simulink model "Code_Gen_Model"  (R2023b)
settings: Solver=FixedStepDiscrete  StartTime=0.0  StopTime=inf  FixedStep=t_sample  RelTol=1e-3
settings Model: Creator=FIRSTMentor  LastModifiedBy=USER
settings OptimizationCC: DefaultParameterBehavior=Inlined  StrengthReduction=on  PassReuseOutputArgsAs=Individual arguments  ZeroExternalMemoryAtStartup=off  ZeroInternalMemoryAtStartup=off  OptimizeBlockOrder=speed  OptimizationPriority=Speed  OptimizationCustomize=off  MultiThreadedLoops=on  EfficientTunableParamExpr=on
settings DebuggingCC: MergeDetectMultiDrivingBlocksExec=none  ParameterTunabilityLossMsg=error
settings HardwareCC: ProdBitPerPointer=32  ProdBitPerSizeT=32  ProdBitPerPtrDiffT=32  ProdLargestAtomicInteger=Long  ProdWordSize=32  ProdHWDeviceType=ARM Compatible->ARM 7
settings ModelReferenceCC: PropagateSignalLabelsOutOfModel=off
settings SFSimCC: MATLABDynamicMemAlloc=off
settings RTWCC: Description=Embedded Coder  SystemTargetFile=ert.tlc  GenCodeOnly=on  TemplateMakefile=ert_default_tmf  Toolchain=MinGW64 | gmake (64-bit Windows)
settings CodeAppCC: ForceParamTrailComments=on  IgnoreCustomStorageClasses=off  OperatorAnnotations=on  SimulinkDataObjDesc=on  SFDataObjDesc=on  InsertBlockDesc=on
settings ERTTargetCC: TargetLangStandard=C99 (ISO)  SupportVariableSizeSignals=on  ParenthesesLevel=Maximum  InlinedParameterPlacement=NonHierarchical  ERTCustomFileTemplate=example_file_process.tlc

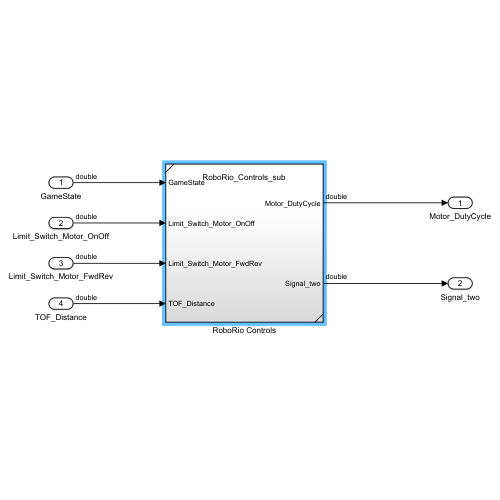
[thumbnail: Simulink's stored preview of the top-level diagram]
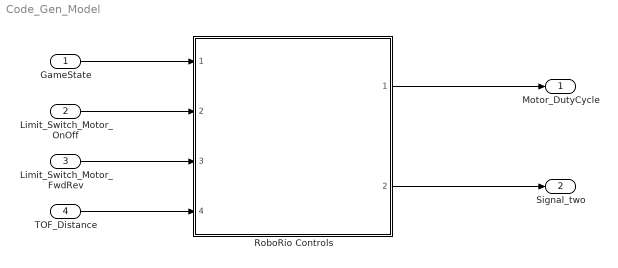
== system Code_Gen_Model ==
  GameState : Inport
  Limit_Switch_Motor_OnOff : Inport  Port=2
  Limit_Switch_Motor_FwdRev : Inport  Port=3
  TOF_Distance : Inport  Port=4
  RoboRio Controls : Subsystem  ReferencedSubsystem=RoboRio_Controls_sub
  Motor_DutyCycle : Outport
  Signal_two : Outport  Port=2
  wires:
  GameState/1 -> RoboRio Controls/1
  RoboRio Controls/1 -> Motor_DutyCycle/1
  RoboRio Controls/2 -> Signal_two/1
  Limit_Switch_Motor_OnOff/1 -> RoboRio Controls/2
  Limit_Switch_Motor_FwdRev/1 -> RoboRio Controls/3
  TOF_Distance/1 -> RoboRio Controls/4
